simulink model "x64_15l_gonly"  (R2012b)
settings: Solver=VariableStepDiscrete  SolverMode=SingleTasking  StartTime=0.0  StopTime=10.0  RelTol=1e-3
undefined symbols (not defined in the file): gcbh, pfb_coeff_gen_calc, ROACH, xlBlockLoadCallback
libraries: xbsIndex_r4 x10760, casper_library_misc x122, casper_library_delays x52, ox_lib x14, xrbsComm_r4 x8, xps_library x8
(part 2 of 128)

== system x64_15l_gonly/a ==
  sync : Inport
  in0 : Inport  Port=2
  in1 : Inport  Port=3
  in2 : Inport  Port=4
  in3 : Inport  Port=5
  in4 : Inport  Port=6
  in5 : Inport  Port=7
  in6 : Inport  Port=8
  in7 : Inport  Port=9
  c : xbsIndex_r4/Constant  const=1  gui_display_data_type=Fixed-point  arith_type=Boolean  n_bits=16  bin_pt=14  preci_type=Single  exp_width=8  frac_width=24  explicit_period=on  period=1  equ=P=C  opselect=C  inp2=PCIN>>17  opr=+  inp1=P  carry=CIN  dbl_ovrd=off  block_type=constant
      settings: block_version=11.4
  r : Subsystem  AncestorBlock=casper_library_reorder/reorder  mask(reorder){map=[0          4          8         12         16         20         24         28         32         36         40         44         48         52         56         60         64         68         72         76         80         84         88         92         96        100        104        108        112        116        120        124        128        132        136        140        144        148        152        156        160        164        168        172        176        180        184        188        192        196        200        204        208        212        216        220        224        228        232        236        240        244        248        252        256        260        264        268        272        276        280        284        288        292        296        300        304        308        312        316        320        324        328        332        336        340        344        348        352        356        360        364        368        372        376        380        384        388        392        396        400        404        408        412        416        420        424        428        432        436        440        444        448        452        456        460        464        468        472        476        480        484        488        492        496        500        504        508        512        516        520        524        528        532        536        540        544        548        552        556        560        564        568        572        576        580        584        588        592        596        600        604        608        612        616        620        624        628        632        636        640        644        648        652        656        660        664        668        672        676        680        684        688        692        696        700        704        708        712        716        720        724        728        732        736        740        744        748        752        756        760        764        768        772        776        780        784        788        792        796        800        804        808        812        816        820        824        828        832        836        840        844        848        852        856        860        864        868        872        876        880        884        888        892        896        900        904        908        912        916        920        924        928        932        936        940        944        948        952        956        960        964        968        972        976        980        984        988        992        996       1000       1004       1008       1012       1016       1020       1024       1028       1032       1036       1040       1044       1048       1052       1056       1060       1064       1068       1072       1076       1080       1084       1088       1092       1096       1100       1104       1108       1112       1116       1120       1124       1128       1132       1136       1140       1144       1148       1152       1156       1160       1164       1168       1172       1176       1180       1184       1188       1192       1196       1200       1204       1208       1212       1216       1220       1224       1228       1232       1236       1240       1244       1248       1252       1256       1260       1264       1268       1272       1276       1280       1284       1288       1292       1296       1300       1304       1308       1312       1316       1320       1324       1328       1332       1336       1340       1344       1348       1352       1356       1360       1364       1368       1372       1376       1380       1384       1388       1392       1396       1400       1404       1408       1412       1416       1420       1424       1428       1432       1436       1440       1444       1448       1452 ...(+86104 chars)], n_bits=0, n_inputs=8, bram_latency=2, map_latency=0, fanout_latency=0, double_buffer=0, bram_map=off}
      mask prompts: map "Output Order:"; n_bits "Data width in"; n_inputs "Number of inputs"; bram_latency "BRAM Latency"; map_latency "Map Latency"; fanout_latency "Fanout latency"; double_buffer "Double Buffer"; bram_map "Use BlockRAM for Map"
      mask init: same as x64_15l_gonly/reorder
      settings: AttributesFormatString=order=13
      mask Help: eval('xlWeb(''http://casper.berkeley.edu/wiki/Reorder'')')
  t : Terminator
  sync_out : Outport
  Out0 : Outport  Port=2
  Out1 : Outport  Port=3
  Out2 : Outport  Port=4
  Out3 : Outport  Port=5
  Out4 : Outport  Port=6
  Out5 : Outport  Port=7
  Out6 : Outport  Port=8
  Out7 : Outport  Port=9
  wires:
  r/10(dout7) -> Out7/1
  r/9(dout6) -> Out6/1
  r/8(dout5) -> Out5/1
  r/7(dout4) -> Out4/1
  r/6(dout3) -> Out3/1
  r/5(dout2) -> Out2/1
  r/4(dout1) -> Out1/1
  r/3(dout0) -> Out0/1
  r/2(valid) -> t/1
  r/1(sync_out) -> sync_out/1
  in7/1 -> r/10(din7)
  in6/1 -> r/9(din6)
  in5/1 -> r/8(din5)
  in4/1 -> r/7(din4)
  in3/1 -> r/6(din3)
  in2/1 -> r/5(din2)
  in1/1 -> r/4(din1)
  in0/1 -> r/3(din0)
  sync/1 -> r/1(sync)
  c/1 -> r/2(en)
